simulink model "s_adrc_1"  (R2020b)
settings: Solver=VariableStepAuto  StartTime=0.0  StopTime=10
settings Model: Creator=Amir  LastModifiedBy=Amir
settings DataIOCC: ReturnWorkspaceOutputs=off

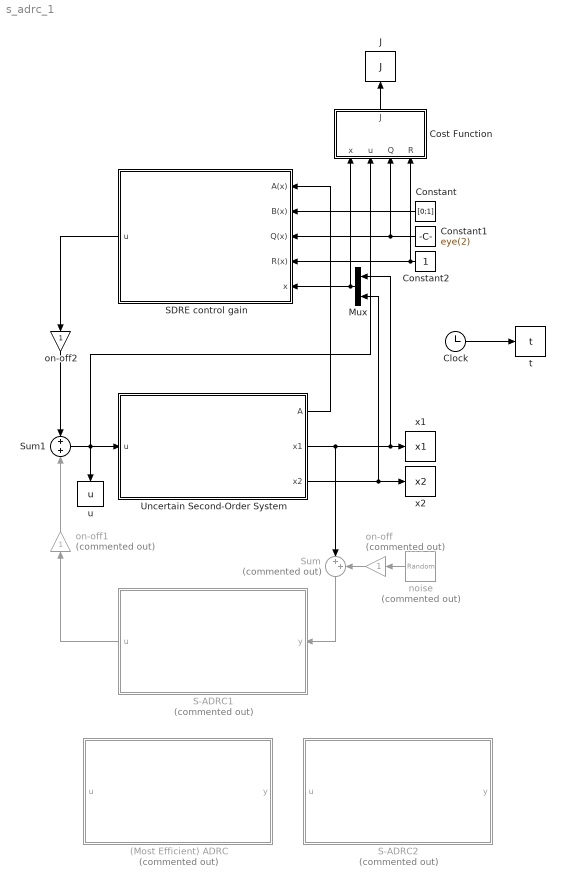
== system s_adrc_1 ==
  (Most Efficient) ADRC : Subsystem  Commented=on  mask{alpha1=3, alpha2=3, alpha3=1, epsilon=0.05, xhat0=[1;2;0], p=2, rho=3^0.5, beta=17.4, delta=(17.4)^0.5, deltap=1e+6}
      mask prompts: xhat0 "xhat(0):"; deltap "delta_prime:"
      mask DialogControl ParameterGroupVar Prompt: LESO Parameters
      mask DialogControl ParameterGroupVar_copy Prompt: Controller Parameters
      mask DialogControl ParameterGroupVar_copy_copy Prompt: Thresholds
  Clock : Clock
  Constant : Constant  Value=[0;1]
  Constant1 : Constant  Value=eye(2)
  Constant2 : Constant
  Cost Function : Subsystem
  J : ToWorkspace  VariableName=J  SampleTime=-1
      settings: Save2DSignal=2-D array (concatenate along first dimension)
  Mux : Mux  Inputs=2
  S-ADRC1 : Subsystem  Commented=on  mask{alpha1=3, alpha2=3, alpha3=1, epsilon=0.05, xhat0=[1;2;0], p=2, rho=1, beta=9, delta=1e+6, deltap=1e+6}
      mask prompts: xhat0 "xhat(0):"; deltap "delta_prime:"
      mask DialogControl ParameterGroupVar Prompt: LESO Parameters
      mask DialogControl ParameterGroupVar_copy Prompt: Controller Parameters
      mask DialogControl ParameterGroupVar_copy_copy Prompt: Thresholds
  S-ADRC2 : Subsystem  Commented=on  mask{alpha1=3, alpha2=3, alpha3=1, epsilon=0.05, xhat0=[1;2;0], p=2, rho=3^0.5, beta=1+2*(2+3^0.5), delta=1e+6, deltap=1e+6}
      mask prompts: xhat0 "xhat(0):"; deltap "delta_prime:"
      mask DialogControl ParameterGroupVar Prompt: LESO Parameters
      mask DialogControl ParameterGroupVar_copy Prompt: Controller Parameters
      mask DialogControl ParameterGroupVar_copy_copy Prompt: Thresholds
  SDRE control gain : Subsystem  mask{n=2, m=1}
      mask prompts: n "Dimension of state vector (x):"; m "Dimension of control input vector (u):"
      mask Help:
      | Introduction:
      | 
      | The state-dependent Riccati equation (SDRE) control technique is a suboptimal controller for systems in the form of dx/dt=f(x)+B(x)*u that can be written as dx/dt=A(x)*x+B(x)*u where A(x) is the state-dependent coefficient (SDC) matrix that satisfies A(x)*x=f(x).
      | The closed-loop response of a nonlinear system under an SDRE controller converges to the optimal trajectory corresponding to the quadratic cost function dJ/dt=x'*Q(x)*x+u'*R(x)*u.
      | The SDRE controller is defined as u=K(x)*x where K(x) is the SDRE controller gain.
      | 
      | Inputs:
      | 
      | 1- The SDC matrix: A(x)
      | 2- Input gain: B(x)
      | 3- Cost function weight for state variables: Q(x)
      | 4- Cost function weight for control input: R(x)
      | 
      | Output:
      | 
      | 1- SDRE controller gain: K(x)
      mask DialogControl DescGroupVar_copy Prompt: SDRE Controller
      mask DialogControl DescTextVar_copy_copy Prompt: This block calculates the controller obtained by the SDRE scheme.
      mask DialogControl Container13 Prompt: Parameters
      mask DialogControl DescGroupVar Prompt: System Dimension
      mask DialogControl Container13_copy Prompt: Help
      mask DialogControl DescGroupVar_copy_copy Prompt: Introduction
      mask DialogControl DescTextVar_copy_copy_copy_copy Prompt: The state-dependent Riccati equation (SDRE) control technique is a suboptimal controller for systems in the form of dx/dt=f(x)+B(x)*u that can be written as dx/dt=A(x)*x+B(x)*u where A(x) is the state-dependent coefficient (SDC) matrix that satisfies A(x)*x=f(x).
      mask DialogControl DescTextVar_copy_copy_copy_copy_copy Prompt: The closed-loop response of a nonlinear system under an SDRE controller converges to the optimal trajectory corresponding to the quadratic cost function dJ/dt=x'*Q(x)*x+u'*R(x)*u.
      mask DialogControl DescTextVar_copy_copy_copy_copy_copy_copy Prompt: The SDRE controller is defined as u=K(x)*x where K(x) is the SDRE controller gain.
      mask DialogControl ParameterGroupVar_copy_copy_copy Prompt: Inputs
      mask DialogControl Control3_copy Prompt: 1- The SDC matrix: A(x)
      mask DialogControl Control5_copy Prompt: 2- Input gain: B(x)
      mask DialogControl Control6_copy Prompt: 3- Cost function weight for state variables: Q(x)
      mask DialogControl Control7_copy Prompt: 4- Cost function weight for control input: R(x)
      mask DialogControl ParameterGroupVar_copy_copy_copy_copy Prompt: Output
      mask DialogControl Control4_copy_copy Prompt: 1- SDRE controller gain: K(x)
      mask DialogControl Container19 Prompt: About
      mask DialogControl Control4_copy_copy_copy Prompt: Refer to the following link for the latest releases and more stuff about SDRE control technique:
      mask DialogControl Control8 Prompt: https://github.com/a-shakouri/SDRE_controller
      mask DialogControl Control8 Callback: web https://github.com/a-shakouri/SDRE_controller
      mask Display: fprintf('SDRE Controller')
  Sum : Sum  Commented=on  Inputs=|++
  Sum1 : Sum  Inputs=+|+
  Uncertain Second-Order System : Subsystem  mask{x0=[1;1]}
      mask prompts: x0 "x(0):"
  noise : RandomNumber  Commented=on  Variance=(0.01)^2  SampleTime=1e-4
  on-off : Gain  Commented=on
  on-off1 : Gain  Commented=on
  on-off2 : Gain
  t : ToWorkspace  VariableName=t  SampleTime=-1
      settings: Save2DSignal=2-D array (concatenate along first dimension)
  u : ToWorkspace  VariableName=u  SampleTime=-1
      settings: Save2DSignal=2-D array (concatenate along first dimension)
  x1 : ToWorkspace  VariableName=x1  SampleTime=-1
      settings: Save2DSignal=2-D array (concatenate along first dimension)
  x2 : ToWorkspace  VariableName=x2  SampleTime=-1
      settings: Save2DSignal=2-D array (concatenate along first dimension)
  wires:
  S-ADRC1/1(u) -> on-off1/1
  Uncertain Second-Order System/3(x2) -> x2/1, Mux/2
  Clock/1 -> t/1
  Uncertain Second-Order System/2(x1) -> Mux/1, x1/1, Sum/1
  Sum/1 -> S-ADRC1/1(y)
  noise/1 -> on-off/1
  on-off/1 -> Sum/2
  Uncertain Second-Order System/1(A) -> SDRE control gain/1(A(x))
  Mux/1 -> SDRE control gain/5(x), Cost Function/1(x)
  Constant/1 -> SDRE control gain/2(B(x))
  Constant1/1 -> Cost Function/3(Q), SDRE control gain/3(Q(x))
  Constant2/1 -> SDRE control gain/4(R(x)), Cost Function/4(R)
  on-off1/1 -> Sum1/2
  SDRE control gain/1(u) -> on-off2/1
  Sum1/1 -> Cost Function/2(u), u/1, Uncertain Second-Order System/1(u)
  on-off2/1 -> Sum1/1
  Cost Function/1(J) -> J/1

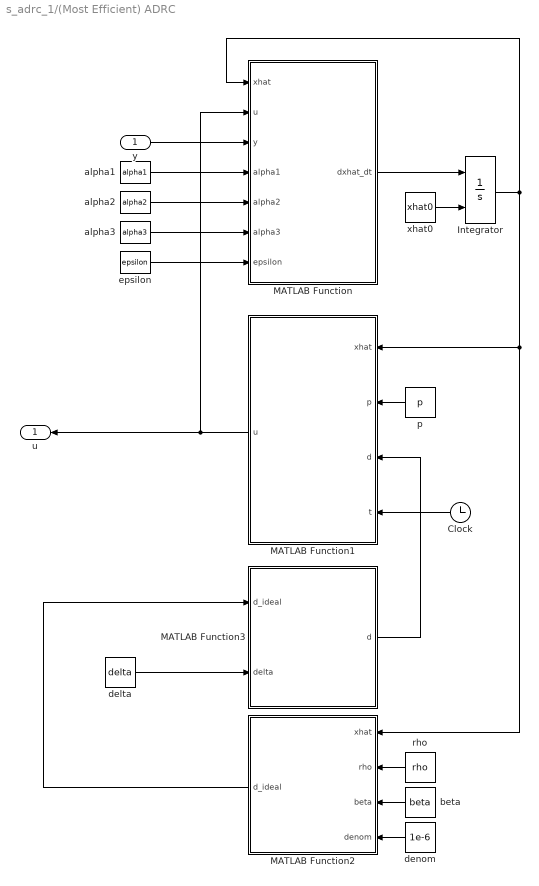
== system s_adrc_1/(Most Efficient) ADRC ==
  y : Inport
  Clock : Clock
  Integrator : Integrator  InitialConditionSource=external
  MATLAB Function : MATLAB Function  TreatAsAtomicUnit=on
  MATLAB Function1 : MATLAB Function  TreatAsAtomicUnit=on
  MATLAB Function2 : MATLAB Function  TreatAsAtomicUnit=on
  MATLAB Function3 : MATLAB Function  TreatAsAtomicUnit=on
  alpha1 : Constant  Value=alpha1
  alpha2 : Constant  Value=alpha2
  alpha3 : Constant  Value=alpha3
  beta : Constant  Value=beta
  delta : Constant  Value=delta
  denom : Constant  Value=1e-6
  epsilon : Constant  Value=epsilon
  p : Constant  Value=p
  rho : Constant  Value=rho
  xhat0 : Constant  Value=xhat0
  u : Outport
  wires:
  Integrator/1 -> MATLAB Function2/1(xhat), MATLAB Function1/1(xhat), MATLAB Function/1(xhat)
  MATLAB Function/1(dxhat_dt) -> Integrator/1
  xhat0/1 -> Integrator/2
  alpha1/1 -> MATLAB Function/4(alpha1)
  alpha2/1 -> MATLAB Function/5(alpha2)
  alpha3/1 -> MATLAB Function/6(alpha3)
  epsilon/1 -> MATLAB Function/7(epsilon)
  y/1 -> MATLAB Function/3(y)
  MATLAB Function1/1(u) -> MATLAB Function/2(u), u/1
  p/1 -> MATLAB Function1/2(p)
  rho/1 -> MATLAB Function2/2(rho)
  beta/1 -> MATLAB Function2/3(beta)
  MATLAB Function3/1(d) -> MATLAB Function1/3(d)
  delta/1 -> MATLAB Function3/2(delta)
  MATLAB Function2/1(d_ideal) -> MATLAB Function3/1(d_ideal)
  denom/1 -> MATLAB Function2/4(denom)
  Clock/1 -> MATLAB Function1/4(t)

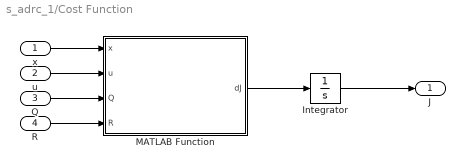
== system s_adrc_1/Cost Function ==
  x : Inport
  u : Inport  Port=2
  Q : Inport  Port=3
  R : Inport  Port=4
  Integrator : Integrator
  MATLAB Function : MATLAB Function  TreatAsAtomicUnit=on
  J : Outport
  wires:
  x/1 -> MATLAB Function/1(x)
  u/1 -> MATLAB Function/2(u)
  Q/1 -> MATLAB Function/3(Q)
  R/1 -> MATLAB Function/4(R)
  MATLAB Function/1(dJ) -> Integrator/1
  Integrator/1 -> J/1

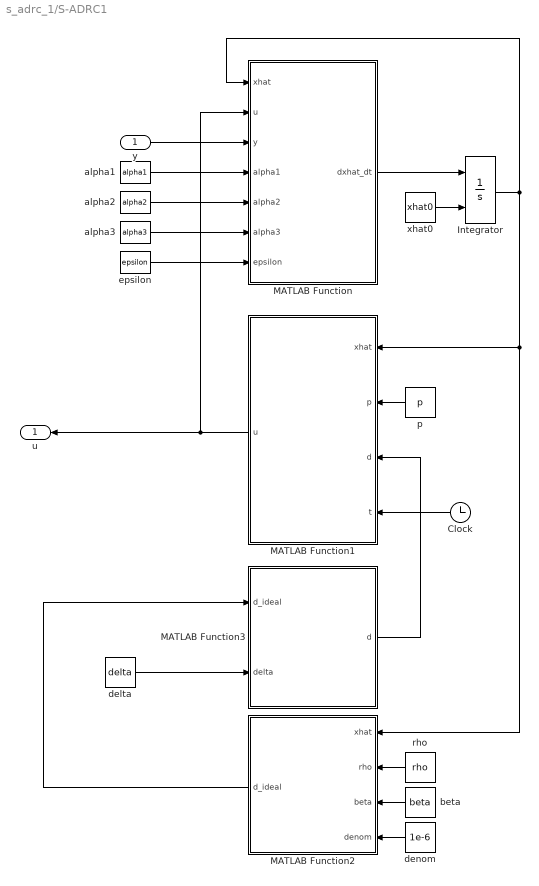
== system s_adrc_1/S-ADRC1 ==
  y : Inport
  Clock : Clock
  Integrator : Integrator  InitialConditionSource=external
  MATLAB Function : MATLAB Function  TreatAsAtomicUnit=on
  MATLAB Function1 : MATLAB Function  TreatAsAtomicUnit=on
  MATLAB Function2 : MATLAB Function  TreatAsAtomicUnit=on
  MATLAB Function3 : MATLAB Function  TreatAsAtomicUnit=on
  alpha1 : Constant  Value=alpha1
  alpha2 : Constant  Value=alpha2
  alpha3 : Constant  Value=alpha3
  beta : Constant  Value=beta
  delta : Constant  Value=delta
  denom : Constant  Value=1e-6
  epsilon : Constant  Value=epsilon
  p : Constant  Value=p
  rho : Constant  Value=rho
  xhat0 : Constant  Value=xhat0
  u : Outport
  wires:
  Integrator/1 -> MATLAB Function2/1(xhat), MATLAB Function1/1(xhat), MATLAB Function/1(xhat)
  MATLAB Function/1(dxhat_dt) -> Integrator/1
  xhat0/1 -> Integrator/2
  alpha1/1 -> MATLAB Function/4(alpha1)
  alpha2/1 -> MATLAB Function/5(alpha2)
  alpha3/1 -> MATLAB Function/6(alpha3)
  epsilon/1 -> MATLAB Function/7(epsilon)
  y/1 -> MATLAB Function/3(y)
  MATLAB Function1/1(u) -> MATLAB Function/2(u), u/1
  p/1 -> MATLAB Function1/2(p)
  rho/1 -> MATLAB Function2/2(rho)
  beta/1 -> MATLAB Function2/3(beta)
  MATLAB Function3/1(d) -> MATLAB Function1/3(d)
  delta/1 -> MATLAB Function3/2(delta)
  MATLAB Function2/1(d_ideal) -> MATLAB Function3/1(d_ideal)
  denom/1 -> MATLAB Function2/4(denom)
  Clock/1 -> MATLAB Function1/4(t)

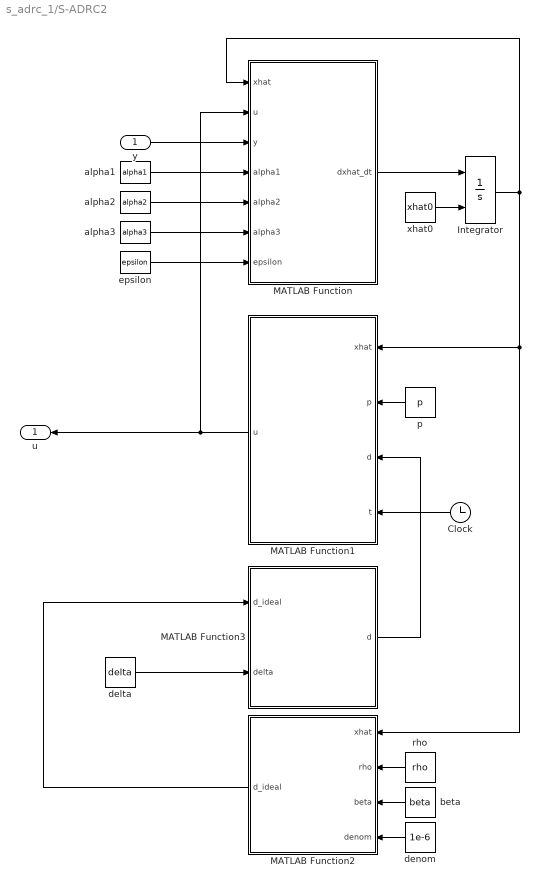
== system s_adrc_1/S-ADRC2 ==
  y : Inport
  Clock : Clock
  Integrator : Integrator  InitialConditionSource=external
  MATLAB Function : MATLAB Function  TreatAsAtomicUnit=on
  MATLAB Function1 : MATLAB Function  TreatAsAtomicUnit=on
  MATLAB Function2 : MATLAB Function  TreatAsAtomicUnit=on
  MATLAB Function3 : MATLAB Function  TreatAsAtomicUnit=on
  alpha1 : Constant  Value=alpha1
  alpha2 : Constant  Value=alpha2
  alpha3 : Constant  Value=alpha3
  beta : Constant  Value=beta
  delta : Constant  Value=delta
  denom : Constant  Value=1e-6
  epsilon : Constant  Value=epsilon
  p : Constant  Value=p
  rho : Constant  Value=rho
  xhat0 : Constant  Value=xhat0
  u : Outport
  wires:
  Integrator/1 -> MATLAB Function2/1(xhat), MATLAB Function1/1(xhat), MATLAB Function/1(xhat)
  MATLAB Function/1(dxhat_dt) -> Integrator/1
  xhat0/1 -> Integrator/2
  alpha1/1 -> MATLAB Function/4(alpha1)
  alpha2/1 -> MATLAB Function/5(alpha2)
  alpha3/1 -> MATLAB Function/6(alpha3)
  epsilon/1 -> MATLAB Function/7(epsilon)
  y/1 -> MATLAB Function/3(y)
  MATLAB Function1/1(u) -> MATLAB Function/2(u), u/1
  p/1 -> MATLAB Function1/2(p)
  rho/1 -> MATLAB Function2/2(rho)
  beta/1 -> MATLAB Function2/3(beta)
  MATLAB Function3/1(d) -> MATLAB Function1/3(d)
  delta/1 -> MATLAB Function3/2(delta)
  MATLAB Function2/1(d_ideal) -> MATLAB Function3/1(d_ideal)
  denom/1 -> MATLAB Function2/4(denom)
  Clock/1 -> MATLAB Function1/4(t)

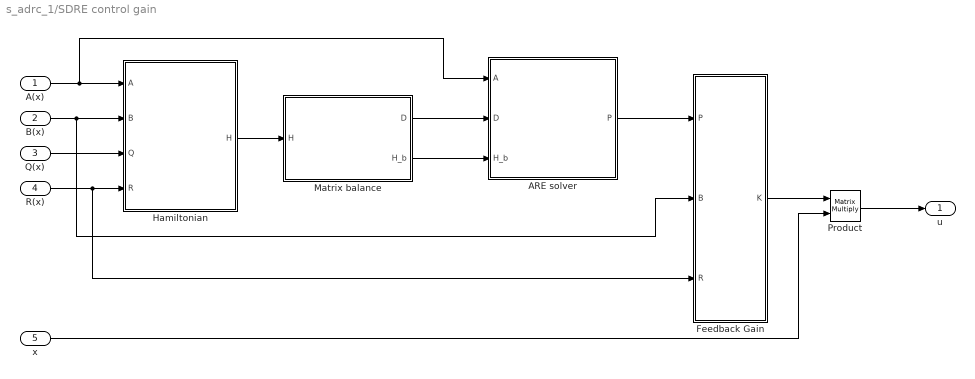
== system s_adrc_1/SDRE control gain ==
  A(x) : Inport
  B(x) : Inport  Port=2
  Q(x) : Inport  Port=3
  R(x) : Inport  Port=4
  x : Inport  Port=5
  ARE solver : MATLAB Function  TreatAsAtomicUnit=on
  Feedback Gain : MATLAB Function  TreatAsAtomicUnit=on
  Hamiltonian : MATLAB Function  TreatAsAtomicUnit=on
  Matrix balance : MATLAB Function  TreatAsAtomicUnit=on
  Product : Product  Multiplication=Matrix(*)
  u : Outport
  wires:
  Hamiltonian/1(H) -> Matrix balance/1(H)
  A(x)/1 -> Hamiltonian/1(A), ARE solver/1(A)
  Matrix balance/2(H_b) -> ARE solver/3(H_b)
  Matrix balance/1(D) -> ARE solver/2(D)
  ARE solver/1(P) -> Feedback Gain/1(P)
  B(x)/1 -> Feedback Gain/2(B), Hamiltonian/2(B)
  Q(x)/1 -> Hamiltonian/3(Q)
  R(x)/1 -> Feedback Gain/3(R), Hamiltonian/4(R)
  Feedback Gain/1(K) -> Product/1
  Product/1 -> u/1
  x/1 -> Product/2

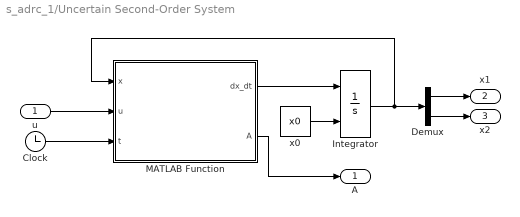
== system s_adrc_1/Uncertain Second-Order System ==
  u : Inport
  Clock : Clock
  Demux : Demux  Outputs=2
  Integrator : Integrator  InitialConditionSource=external
  MATLAB Function : MATLAB Function  TreatAsAtomicUnit=on
  x0 : Constant  Value=x0
  A : Outport
  x1 : Outport  Port=2
  x2 : Outport  Port=3
  wires:
  Integrator/1 -> Demux/1, MATLAB Function/1(x)
  MATLAB Function/1(dx_dt) -> Integrator/1
  Demux/1 -> x1/1
  Demux/2 -> x2/1
  u/1 -> MATLAB Function/2(u)
  Clock/1 -> MATLAB Function/3(t)
  x0/1 -> Integrator/2
  MATLAB Function/2(A) -> A/1

== matlab function s_adrc_1/Cost Function/MATLAB Function ==
  data: x input; u input; dJ output; Q input; R input
function dJ  = cost_gen(x,u,Q,R)

dJ=0.5*(x'*Q*x+u'*R*u);

== matlab function s_adrc_1/S-ADRC1/MATLAB Function ==
  data: xhat input; u input; y input; dxhat_dt output; alpha1 input; alpha2 input; alpha3 input; epsilon input
function dxhat_dt = LESO(xhat,u,y,alpha1,alpha2,alpha3,epsilon)

g=1;

dxhat_dt=[xhat(2)+(alpha1/epsilon)*(y-xhat(1))
          xhat(3)+(alpha2/epsilon^2)*(y-xhat(1))+g*u
          (alpha3/epsilon^3)*(y-xhat(1))];

== matlab function s_adrc_1/S-ADRC1/MATLAB Function1 ==
  data: xhat input; p input; d input; u output; t input
function u = Controller(xhat,p,d,t)

% d=4.2;

u=-p*xhat(1)-d*xhat(2)-xhat(3);

if t<0
    
    u=0;
    
end

== matlab function s_adrc_1/S-ADRC1/MATLAB Function2 ==
  data: xhat input; rho input; beta input; d_ideal output; denom input
function d_ideal = d_gen(xhat,rho,beta,denom)

d_ideal=sqrt(((xhat(3)-rho*xhat(1))/(xhat(2)+denom))^2+beta);

== matlab function s_adrc_1/S-ADRC1/MATLAB Function3 ==
  data: d_ideal input; d output; delta input
function d = d_gen(d_ideal,delta)

if d_ideal>delta
    
    d=delta;
    
else

d = d_ideal;

end

== matlab function s_adrc_1/S-ADRC2/MATLAB Function ==
  data: xhat input; u input; y input; dxhat_dt output; alpha1 input; alpha2 input; alpha3 input; epsilon input
function dxhat_dt = LESO(xhat,u,y,alpha1,alpha2,alpha3,epsilon)

g=1;

dxhat_dt=[xhat(2)+(alpha1/epsilon)*(y-xhat(1))
          xhat(3)+(alpha2/epsilon^2)*(y-xhat(1))+g*u
          (alpha3/epsilon^3)*(y-xhat(1))];

== matlab function s_adrc_1/(Most Efficient) ADRC/MATLAB Function ==
  data: xhat input; u input; y input; dxhat_dt output; alpha1 input; alpha2 input; alpha3 input; epsilon input
function dxhat_dt = LESO(xhat,u,y,alpha1,alpha2,alpha3,epsilon)

g=1;

dxhat_dt=[xhat(2)+(alpha1/epsilon)*(y-xhat(1))
          xhat(3)+(alpha2/epsilon^2)*(y-xhat(1))+g*u
          (alpha3/epsilon^3)*(y-xhat(1))];

== matlab function s_adrc_1/S-ADRC2/MATLAB Function1 ==
  data: xhat input; p input; d input; u output; t input
function u = Controller(xhat,p,d,t)

% d=4.2;

u=-p*xhat(1)-d*xhat(2)-xhat(3);

if t<0
    
    u=0;
    
end

== matlab function s_adrc_1/S-ADRC2/MATLAB Function2 ==
  data: xhat input; rho input; beta input; d_ideal output; denom input
function d_ideal = d_gen(xhat,rho,beta,denom)

d_ideal=sqrt(((xhat(3)-rho*xhat(1))/(xhat(2)+denom))^2+beta);

== matlab function s_adrc_1/S-ADRC2/MATLAB Function3 ==
  data: d_ideal input; d output; delta input
function d = d_gen(d_ideal,delta)

if d_ideal>delta
    
    d=delta;
    
else

d = d_ideal;

end

== matlab function s_adrc_1/Uncertain Second-Order System/MATLAB Function ==
  data: x input; u input; dx_dt output; t input; A output
function [dx_dt,A] = dyn(x,u,t)

f=exp(sin(t))*x(1)+t*cos(t^2)*x(2);%(1+exp(-t))*sin(x(1));%-x(1)+0.1*(1-x(1)^2)*x(2);%

A=[0           1
   exp(sin(t)) t*cos(t^2)];



% A=[0 1
%    (1+exp(-t))*sin(x(1))/x(1) 0];

% A=[0 1
%    3^0.5 ((1+exp(-t))*sin(x(1))-3^0.5*x(1))/x(2)];
 
% A=[0 1
%    (exp(-t))*sin(x(1))/x(1) (1)*sin(x(1))/x(2)];
 
% A=[0 1
%    (1)*sin(x(1))/x(1) (exp(-t))*sin(x(1))/x(2)];

dx_dt = [x(2)
         f+u];

== matlab function s_adrc_1/(Most Efficient) ADRC/MATLAB Function1 ==
  data: xhat input; p input; d input; u output; t input
function u = Controller(xhat,p,d,t)

% d=4.2;

u=-p*xhat(1)-d*xhat(2)-xhat(3);

if t<0
    
    u=0;
    
end

== matlab function s_adrc_1/(Most Efficient) ADRC/MATLAB Function2 ==
  data: xhat input; rho input; beta input; d_ideal output; denom input
function d_ideal = d_gen(xhat,rho,beta,denom)

d_ideal=sqrt(((xhat(3)-rho*xhat(1))/(xhat(2)+denom))^2+beta);

== matlab function s_adrc_1/(Most Efficient) ADRC/MATLAB Function3 ==
  data: d_ideal input; d output; delta input
function d = d_gen(d_ideal,delta)

if d_ideal>delta
    
    d=delta;
    
else

d = d_ideal;

end

== matlab function s_adrc_1/SDRE control gain/ARE solver ==
  data: A input size=[n n]; D input size=[2*n 2*n]; H_b input size=[2*n 2*n]; P output size=[n n]
function P = ARE_diag(A, D, H_b)

    n = size(A,1);
    
    P = zeros(n,n);
    
    [T,L] = eig(H_b);
    
    T = D*T;
    
    lambda = diag(L);
    ord_lambda = zeros(1,2*n);
    for k = 1 : 2*n;
        if real(lambda(k)) < 0
            ord_lambda(k) = -1;
        elseif real(lambda(k)) > 0
            ord_lambda(k) = 1;
        else
            %disp('!!!');
        end
    end
    
    [~, ord_index] = sort(ord_lambda, 'descend');

    T_ord = T(:,ord_index);

    T22 = T_ord(n+1:2*n,n+1:2*n);
    T12 = T_ord(1:n,n+1:2*n);
    
    P = real(T22/T12);

== matlab function s_adrc_1/SDRE control gain/Feedback Gain ==
  data: P input size=[n n]; B input size=[n m]; K output size=[m n]; R input size=[m m]
function K  = u_in_gen(P,B,R)

K=-(inv(R))*B'*P;

end

== matlab function s_adrc_1/SDRE control gain/Hamiltonian ==
  data: A input size=[n n]; H output size=[2*n 2*n]; B input size=[n m]; Q input size=[n n]; R input size=[m m]
function H  = Hamilton(A, B, Q, R)
    
H = [A -(B/R)*B'; -Q -A'];

== matlab function s_adrc_1/SDRE control gain/Matrix balance ==
  data: H input size=[2*n 2*n]; D output size=[2*n 2*n]; H_b output size=[2*n 2*n]
function [D, H_b] = matrix_balance(H)
    
% Numerical Recipes p.593 - Balancing (vedi anche articolo James)
% Trasformazione
% D^-1 * A * D = B 
    
A=H;

    n = size(A,1);
    B = A;
    D = eye(n);
    
    RADIX = 2;
    sqrdx = RADIX*RADIX;
    
    done = 0;
    
    while done ~= 1 
        
        done = 1;
        
        for i = 1 : n 
            
            r = 0;
            c = 0;
            
            for j = 1 : n
                if j ~= i 
                    c = c + abs(B(j,i));
                    r = r + abs(B(i,j));
                end
            end
                
            if c ~= 0 && r ~= 0 
                g = r/RADIX;
                f = 1;
                s = c + r;
                
                while (c<g) 
                    f = f*RADIX;
                    c = c*sqrdx;
                end
                
                g = r*RADIX;
                
                while c > g 
                    f = f/RADIX;
                    c = c/sqrdx;
                end
                
                if (c + r)/f < 0.95*s 
                    done = 0;
                    g = 1/f;
                    D(i,i) = D(i,i)*f;

                    for j = 1 : n 
                        B(i,j) = B(i,j)/f; 
                    end
                    
                    for j = 1 : n
                        B(j,i) = B(j,i)*f;
                    end
                end
            end
        end
    end
    
H_b=B;
